simulink model "PositionControl"  (R2020a)
settings: Solver=ode3  StartTime=0.0  StopTime=100.0  FixedStep=Ts  RelTol=1e-3
values from neighbouring files (symbols this model uses):
  refx = 10*rand    [RunPositionControl.m]
  refy = 10*rand    [RunPositionControl.m]
libraries: fuzblock x1, simulink x1
settings Model: Creator=atien  LastModifiedBy=charlie
settings DataIOCC: ReturnWorkspaceOutputs=off

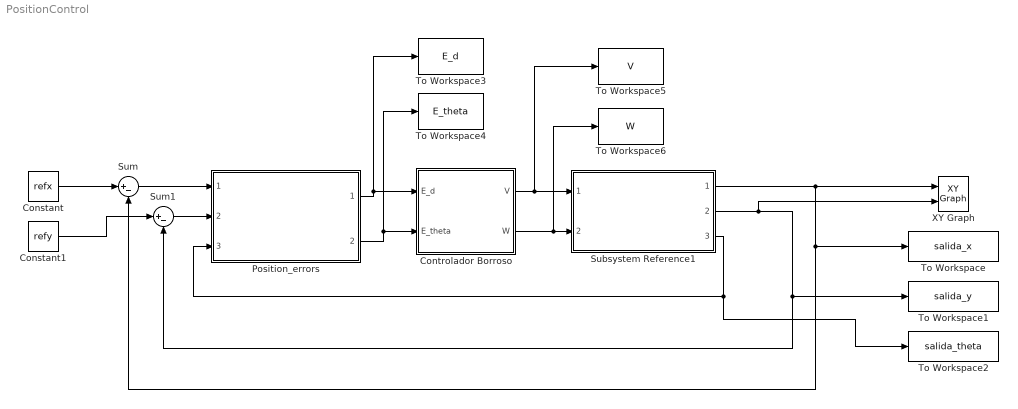
== system PositionControl ==
  Constant : Constant  Value=refx
  Constant1 : Constant  Value=refy
  Controlador Borroso : Subsystem
  Position_errors : Subsystem  ReferencedSubsystem=PositionErrors
  Subsystem Reference1 : Subsystem  ReferencedSubsystem=robot
  Sum : Sum  Inputs=|+-
  Sum1 : Sum  Inputs=|+-
  To Workspace : ToWorkspace  VariableName=salida_x  SaveFormat=Structure With Time  SampleTime=-1
  To Workspace1 : ToWorkspace  VariableName=salida_y  SaveFormat=Structure With Time  SampleTime=-1
  To Workspace2 : ToWorkspace  VariableName=salida_theta  SaveFormat=Structure With Time  SampleTime=-1
  To Workspace3 : ToWorkspace  VariableName=E_d  SaveFormat=Structure With Time  SampleTime=-1
  To Workspace4 : ToWorkspace  VariableName=E_theta  SaveFormat=Structure With Time  SampleTime=-1
  To Workspace5 : ToWorkspace  VariableName=V  SaveFormat=Structure With Time  SampleTime=-1
  To Workspace6 : ToWorkspace  VariableName=W  SaveFormat=Structure With Time  SampleTime=-1
  XY Graph : simulink/Sinks/XY Graph  xmin=-5  xmax=5  ymin=-5  ymax=5  st=-1
  wires:
  Subsystem Reference1/3 -> To Workspace2/1, Position_errors/3
  Controlador Borroso/2(W) -> Subsystem Reference1/2, To Workspace6/1
  Controlador Borroso/1(V) -> To Workspace5/1, Subsystem Reference1/1
  Subsystem Reference1/1 -> To Workspace/1, Sum/2, XY Graph/1
  Constant/1 -> Sum/1
  Sum1/1 -> Position_errors/2
  Sum/1 -> Position_errors/1
  Position_errors/2 -> Controlador Borroso/2(E_theta), To Workspace4/1
  Subsystem Reference1/2 -> XY Graph/2, To Workspace1/1, Sum1/2
  Constant1/1 -> Sum1/1
  Position_errors/1 -> Controlador Borroso/1(E_d), To Workspace3/1

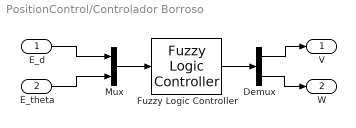
== system PositionControl/Controlador Borroso ==
  E_d : Inport
  E_theta : Inport  Port=2
  Demux : Demux  Outputs=2
  Fuzzy Logic Controller : fuzblock/Fuzzy Logic  Controller  FIS='ControlBorroso.fis'  OutputSampleNumber=101  DataType=double  FuzzifiedInputs=off  RuleFiringStrengths=off  RuleOutputs=off  AggregatedOutputs=off  SimulateUsing=Interpreted execution  OutOfRangeInputValueMessage=warning  NoRuleFiredMessage=warning  EmptyOutputFuzzySetMessage=warning
  Mux : Mux  Inputs=2
  V : Outport
  W : Outport  Port=2
  wires:
  Mux/1 -> Fuzzy Logic Controller/1
  Fuzzy Logic Controller/1 -> Demux/1
  E_d/1 -> Mux/1
  E_theta/1 -> Mux/2
  Demux/1 -> V/1
  Demux/2 -> W/1
